simulink model "sim_real"  (R2016a)
settings: Solver=FixedStepAuto  StartTime=0.0  StopTime=25  RelTol=1e-3
InitFcn:
  | % Parametros
  | clear;
  | alpha1 = 0;
  | alpha2 = 120*pi/180;
  | alpha3 = 240*pi/180;
  | g = 9.8;
  | vs = 6e-10;
  | M = 1.83;
  | l1 = 0.09;
  | l2 = 0.09;
  | l3 = 0.09;
  | r1 = 0.072;
  | r2 = 0.072;
  | r3 = 0.072;
  | kt = 0.0059;
  | kem = 0.0059;
  | N = 19;
  | L = 0.00011;
  | R = 1.71;
  | Jm1 = 3.88e-7;
  | Jm2 = 3.88e-7;
  | Jm3 = 3.88e-7;
  | J1 = 8.1e-4;
  | J2 = 8.1e-4;
  | J3 = 8.1e-4;
  | J = 2.125;
  | eta = 0.83;
  | freq = 1000; % varia entre 2.5kHz e 5Mhz
  | mic = 0.46;
  | mis = 0.46;
  | sigma0 = 100;
  | sigma1 = 0.1;
  | sigma2 = 0.1;
  | 
  | mi = 0.25;
  | b = .1;
  | 
  | % Controlador
  | Kpx = 10;
  | Kix = 25;
  | Kpy = 10;
  | Kiy = 25;
  | Kvphi = 3;
  | Kpphi = 2.25;
  | 
  | kctr = kt*5.4*eta*N/(R*r1)
undefined symbols (not defined in the file or in its folder): magnitude
settings Model: MinMaxOverflowLogging=MinMaxAndOverflow  Creator=Pichau  LastModifiedBy=Pichau
settings DataIOCC: LimitDataPoints=on  MaxDataPoints=100000000  SaveFormat=Array  SignalLoggingSaveFormat=ModelDataLogs
settings OptimizationCC: OptimizeBlockIOStorage=off  BufferReuse=off  GlobalBufferReuse=off  ExpressionFolding=off  LocalBlockOutputs=off  RollThreshold=4
settings DebuggingCC: SaveWithParameterizedLinksMsg=none  UnderspecifiedInitializationDetection=Classic  MergeDetectMultiDrivingBlocksExec=none  SignalResolutionControl=TryResolveAllWithWarning  MultiTaskDSMMsg=warning  MultiTaskCondExecSysMsg=none
settings HardwareCC: ProdBitPerPointer=32  ProdLargestAtomicFloat=None  ProdIntDivRoundTo=Undefined  ProdEndianess=Unspecified  ProdWordSize=32  ProdHWDeviceType=32-bit Generic  TargetUnknown=on
settings ModelReferenceCC: PropagateSignalLabelsOutOfModel=off
settings GRTTargetCC: TargetFcnLib=ansi_tfl_tmw.mat  GeneratePreprocessorConditionals=Use local settings  CombineOutputUpdateFcns=off  GRTInterface=on
settings ConfigComp: CovModelRefEnable=Off

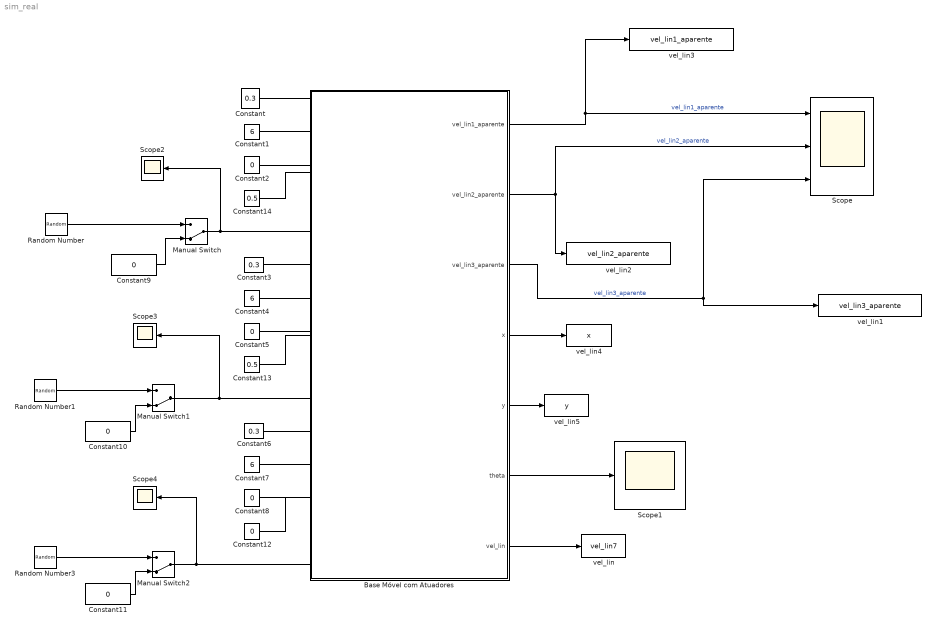
== system sim_real ==
  Base Móvel com Atuadores : Subsystem
  Constant : Constant  Value=0.3
  Constant1 : Constant  Value=6
  Constant{2,5,8..12} (7 alike) : Constant  Value=0
  Constant13 : Constant  Value=0.5
  Constant14 : Constant  Value=0.5
  Constant3 : Constant  Value=0.3
  Constant4 : Constant  Value=6
  Constant6 : Constant  Value=0.3
  Constant7 : Constant  Value=6
  Manual Switch : ManualSwitch  CurrentSetting=0
  Manual Switch1 : ManualSwitch  CurrentSetting=0
  Manual Switch2 : ManualSwitch  CurrentSetting=0
  Random Number : RandomNumber  Variance=0.003  Seed=123123  SampleTime=10
  Random Number1 : RandomNumber  Variance=0.003  Seed=2323  SampleTime=10
  Random Number3 : RandomNumber  Variance=0.003  Seed=55  SampleTime=10
  Scope : Scope  NumInputPorts=3
  Scope{1..4} (4 alike) : Scope
  vel_lin : ToWorkspace  VariableName=vel_lin7  SampleTime=0.01
  vel_lin1 : ToWorkspace  VariableName=vel_lin3_aparente  SampleTime=-1
  vel_lin2 : ToWorkspace  VariableName=vel_lin2_aparente  SampleTime=-1
  vel_lin3 : ToWorkspace  VariableName=vel_lin1_aparente  SampleTime=-1
  vel_lin4 : ToWorkspace  VariableName=x  SampleTime=-1
  vel_lin5 : ToWorkspace  VariableName=y  SampleTime=-1
  wires:
  Constant/1 -> ?
  Constant1/1 -> ?
  Constant2/1 -> ?
  Constant14/1 -> ?
  Constant9/1 -> Manual Switch/2
  Constant3/1 -> ?
  Constant4/1 -> ?
  Constant5/1 -> ?
  Constant13/1 -> ?
  Constant6/1 -> ?
  Constant7/1 -> ?
  Constant8/1 -> ?
  Constant12/1 -> ?
  Base Móvel com Atuadores/7(vel_lin) -> vel_lin/1
  Base Móvel com Atuadores/1(vel_lin1_aparente) -> vel_lin3/1, Scope/1  "vel_lin1_aparente"
  Base Móvel com Atuadores/2(vel_lin2_aparente) -> vel_lin2/1, Scope/2  "vel_lin2_aparente"
  Base Móvel com Atuadores/3(vel_lin3_aparente) -> vel_lin1/1, Scope/3  "vel_lin3_aparente"
  Base Móvel com Atuadores/6(theta) -> Scope1/1
  Base Móvel com Atuadores/5(y) -> vel_lin5/1
  Base Móvel com Atuadores/4(x) -> vel_lin4/1
  Random Number/1 -> Manual Switch/1
  Random Number1/1 -> Manual Switch1/1
  Manual Switch/1 -> Scope2/1
  Constant10/1 -> Manual Switch1/2
  Manual Switch1/1 -> Scope3/1
  Random Number3/1 -> Manual Switch2/1
  Constant11/1 -> Manual Switch2/2
  Manual Switch2/1 -> Scope4/1

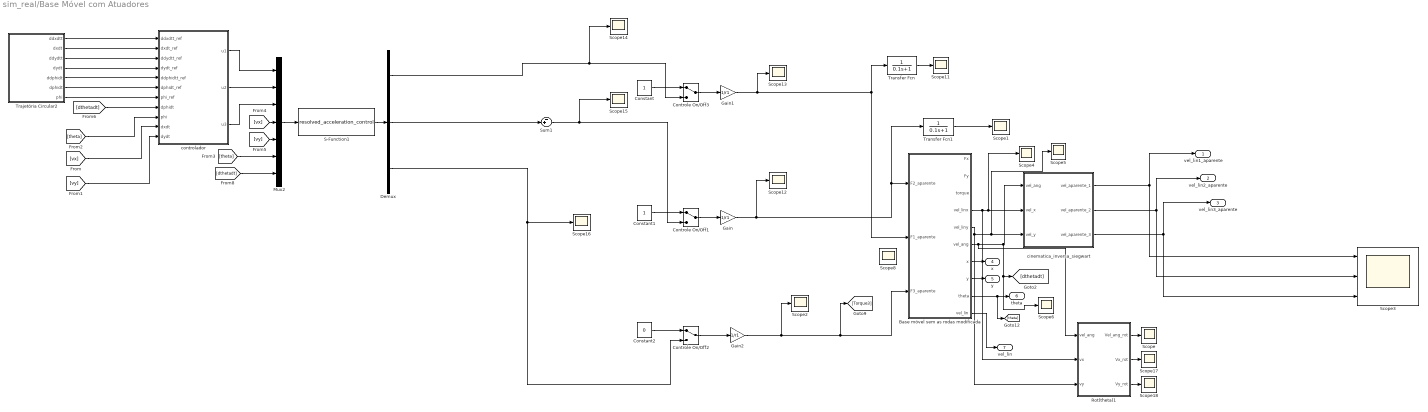
== system sim_real/Base Móvel com Atuadores ==
  Base móvel sem as rodas modificada : Subsystem
  Constant : Constant
  Constant1 : Constant
  Constant2 : Constant  Value=0
  Controle On/Off1 : ManualSwitch
  Controle On/Off2 : ManualSwitch
  Controle On/Off3 : ManualSwitch
  Demux : Demux  Outputs=3
  Gain : Gain  Gain=1/r1
  Gain1 : Gain  Gain=1/r1
  Gain2 : Gain  Gain=1/r1
  Mux2 : Mux  Inputs=7
  Rot(theta)1 : Subsystem
  S-Function1 : S-Function  FunctionName=resolved_acceleration_control  Parameters=r,L,m,J,Jw  SFunctionDeploymentMode=off  EnableBusSupport=off  mask{r=0.072, L=0.09, m=1.83, J=2.125, Jw=8.1e-4}
  Scope{,1..2,4..6,8,11..18} (15 alike) : Scope
  Scope3 : Scope  NumInputPorts=3
  Sum1 : Sum  Inputs=-+|
  Trajetória Circular2 : Subsystem
  Transfer Fcn : TransferFcn  Denominator=[0.1 1]
  Transfer Fcn1 : TransferFcn  Denominator=[0.1 1]
  cinematica_inversa_siegwart : Subsystem
  controlador : Subsystem
  vel_lin1_aparente : Outport
  vel_lin2_aparente : Outport  Port=2
  vel_lin3_aparente : Outport  Port=3
  x : Outport  Port=4
  y : Outport  Port=5
  theta : Outport  Port=6
  vel_lin : Outport  Port=7
  wires:
  cinematica_inversa_siegwart/1(vel_aparente_1) -> vel_lin1_aparente/1, Scope3/1
  Base móvel sem as rodas modificada/4(vel_linx) -> Rot(theta)1/2(vx), Scope4/1, cinematica_inversa_siegwart/2(vel_x)
  Controle On/Off3/1 -> Gain1/1
  cinematica_inversa_siegwart/2(vel_aparente_2) -> vel_lin2_aparente/1, Scope3/2
  cinematica_inversa_siegwart/3(vel_aparente_3) -> vel_lin3_aparente/1, Scope3/3
  Base móvel sem as rodas modificada/7(x) -> x/1
  Base móvel sem as rodas modificada/8(y) -> y/1
  Base móvel sem as rodas modificada/10(vel_lin) -> vel_lin/1
  Base móvel sem as rodas modificada/6(vel_ang) -> Rot(theta)1/1(vel_ang), cinematica_inversa_siegwart/1(vel_ang), [dthetadt], Scope6/1
  Transfer Fcn/1 -> Scope11/1
  Controle On/Off2/1 -> Gain2/1
  Transfer Fcn1/1 -> Scope1/1
  Constant/1 -> Controle On/Off3/1
  Constant1/1 -> Controle On/Off1/1
  Trajetória Circular2/2(dxdt) -> controlador/2(dxdt_ref)
  Trajetória Circular2/6(dphidt) -> controlador/6(dphidt_ref)
  Trajetória Circular2/1(ddxdtt) -> controlador/1(ddxdtt_ref)
  Trajetória Circular2/4(dydt) -> controlador/4(dydt_ref)
  Trajetória Circular2/3(ddydtt) -> controlador/3(ddydtt_ref)
  Trajetória Circular2/7(phi) -> controlador/7(phi_ref)
  Trajetória Circular2/5(ddphidt) -> controlador/5(ddphidtt_ref)
  controlador/1(u1) -> Mux2/1
  controlador/2(u2) -> Mux2/2
  controlador/3(u3) -> Mux2/3
  [vx] -> controlador/10(dxdt)
  [vy] -> controlador/11(dydt)
  [theta] -> controlador/9(phi)
  Mux2/1 -> S-Function1/1
  [theta] -> Mux2/6
  [vx] -> Mux2/4
  [vy] -> Mux2/5
  [dthetadt] -> controlador/8(dphidt)
  [dthetadt] -> Mux2/7
  S-Function1/1 -> Demux/1
  Demux/1 -> Scope14/1, Controle On/Off3/2
  Demux/3 -> Scope16/1, Controle On/Off2/2
  Demux/2 -> Sum1/2
  Controle On/Off1/1 -> Gain/1
  Sum1/1 -> Scope15/1, Controle On/Off1/2
  Base móvel sem as rodas modificada/9(theta) -> [theta], theta/1
  Gain/1 -> Scope12/1, Transfer Fcn1/1, Base móvel sem as rodas modificada/1(F2_aparente)
  Gain1/1 -> Scope13/1, Transfer Fcn/1, Base móvel sem as rodas modificada/2(F1_aparente)
  Gain2/1 -> Scope2/1, Base móvel sem as rodas modificada/3(F3_aparente), [Torque3]
  Rot(theta)1/2(Vx_rot) -> Scope17/1
  Rot(theta)1/3(Vy_rot) -> Scope18/1
  Rot(theta)1/1(Vel_ang_rot) -> Scope/1
  Constant2/1 -> Controle On/Off2/1
  Base móvel sem as rodas modificada/5(vel_liny) -> Rot(theta)1/3(vy), Scope5/1, cinematica_inversa_siegwart/3(vel_y)

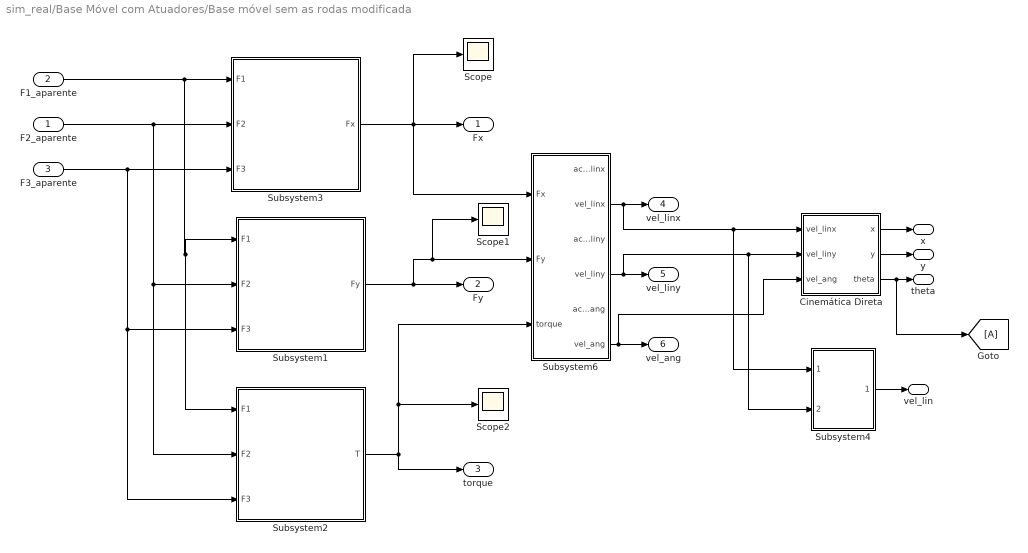
== system sim_real/Base Móvel com Atuadores/Base móvel sem as rodas modificada ==
  F2_aparente : Inport
  F1_aparente : Inport  Port=2
  F3_aparente : Inport  Port=3
  Cinemática Direta : Subsystem
  Scope : Scope
  Scope1 : Scope
  Scope2 : Scope
  Subsystem1 : Subsystem
  Subsystem2 : Subsystem
  Subsystem3 : Subsystem
  Subsystem4 : Subsystem
  Subsystem6 : Subsystem
  Fx : Outport
  Fy : Outport  Port=2
  torque : Outport  Port=3
  vel_linx : Outport  Port=4
  vel_liny : Outport  Port=5
  vel_ang : Outport  Port=6
  x : Outport  Port=7
  y : Outport  Port=8
  theta : Outport  Port=9
  vel_lin : Outport  Port=10
  wires:
  Subsystem3/1(Fx) -> Scope/1, Subsystem6/1(Fx), Fx/1
  Subsystem1/1(Fy) -> Scope1/1, Subsystem6/2(Fy), Fy/1
  F1_aparente/1 -> Subsystem2/1(F1), Subsystem1/1(F1), Subsystem3/1(F1)
  Subsystem6/2(vel_linx) -> vel_linx/1, Cinemática Direta/1(vel_linx), Subsystem4/1(vel_linx)
  Subsystem6/4(vel_liny) -> vel_liny/1, Cinemática Direta/2(vel_liny), Subsystem4/2(vel_liny)
  Subsystem6/6(vel_ang) -> vel_ang/1, Cinemática Direta/3(vel_ang)
  Subsystem2/1(T) -> torque/1, Subsystem6/3(torque), Scope2/1
  Cinemática Direta/1(x) -> x/1
  Cinemática Direta/2(y) -> y/1
  Cinemática Direta/3(theta) -> [A], theta/1
  Subsystem4/1(vel_lin) -> vel_lin/1
  F2_aparente/1 -> Subsystem2/2(F2), Subsystem1/2(F2), Subsystem3/2(F2)
  F3_aparente/1 -> Subsystem2/3(F3), Subsystem1/3(F3), Subsystem3/3(F3)

== system sim_real/Base Móvel com Atuadores/Rot(theta)1 ==
  vel_ang : Inport
  vx : Inport  Port=2
  vy : Inport  Port=3
  Integrator : Integrator
  Subsystem3 : Subsystem
  Subsystem4 : Subsystem
  Vel_ang_rot : Outport
  Vx_rot : Outport  Port=2
  Vy_rot : Outport  Port=3
  wires:
  Integrator/1 -> Subsystem3/1(theta), Subsystem4/1(theta)
  vel_ang/1 -> Integrator/1, Vel_ang_rot/1
  vy/1 -> Subsystem3/3(vy), Subsystem4/3(vy)
  vx/1 -> Subsystem3/2(vx), Subsystem4/2(vx)
  Subsystem4/1(vy_rot) -> Vy_rot/1
  Subsystem3/1(vx_rot) -> Vx_rot/1

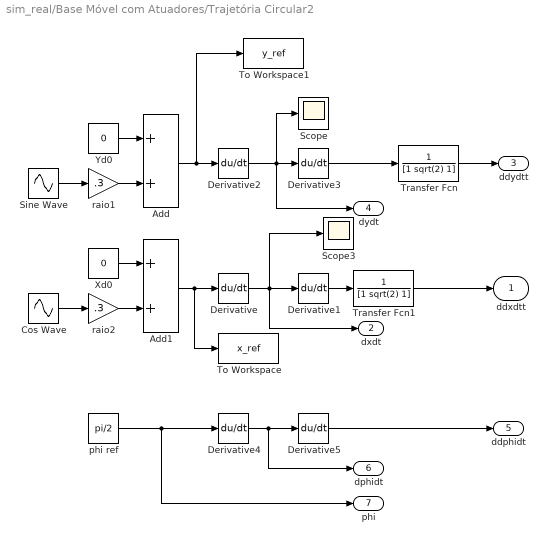
== system sim_real/Base Móvel com Atuadores/Trajetória Circular2 ==
  Add : Sum
  Add1 : Sum
  Cos Wave : Sin  Frequency=0.3  Phase=pi/2  SampleTime=0
  Derivative{,1..5} (6 alike) : Derivative
  Scope : Scope
  Scope3 : Scope
  Sine Wave : Sin  Frequency=0.3  SampleTime=0
  To Workspace : ToWorkspace  VariableName=x_ref  SaveFormat=Timeseries  SampleTime=-1
  To Workspace1 : ToWorkspace  VariableName=y_ref  SaveFormat=Timeseries  SampleTime=-1
  Transfer Fcn : TransferFcn  Denominator=[1 sqrt(2) 1]
  Transfer Fcn1 : TransferFcn  Denominator=[1 sqrt(2) 1]
  Xd0 : Constant  Value=0
  Yd0 : Constant  Value=0
  phi ref : Constant  Value=pi/2
  raio1 : Gain  Gain=.3
  raio2 : Gain  Gain=.3
  ddxdtt : Outport
  dxdt : Outport  Port=2
  ddydtt : Outport  Port=3
  dydt : Outport  Port=4
  ddphidt : Outport  Port=5
  dphidt : Outport  Port=6
  phi : Outport  Port=7
  wires:
  Transfer Fcn1/1 -> ddxdtt/1
  Transfer Fcn/1 -> ddydtt/1
  phi ref/1 -> Derivative4/1, phi/1
  Derivative5/1 -> ddphidt/1
  Derivative4/1 -> Derivative5/1, dphidt/1
  Derivative1/1 -> Transfer Fcn1/1
  Derivative3/1 -> Transfer Fcn/1
  Derivative2/1 -> Derivative3/1, Scope/1, dydt/1
  Derivative/1 -> Scope3/1, Derivative1/1, dxdt/1
  Sine Wave/1 -> raio1/1
  raio1/1 -> Add/2
  Add/1 -> To Workspace1/1, Derivative2/1
  Add1/1 -> To Workspace/1, Derivative/1
  raio2/1 -> Add1/2
  Cos Wave/1 -> raio2/1
  Xd0/1 -> Add1/1
  Yd0/1 -> Add/1

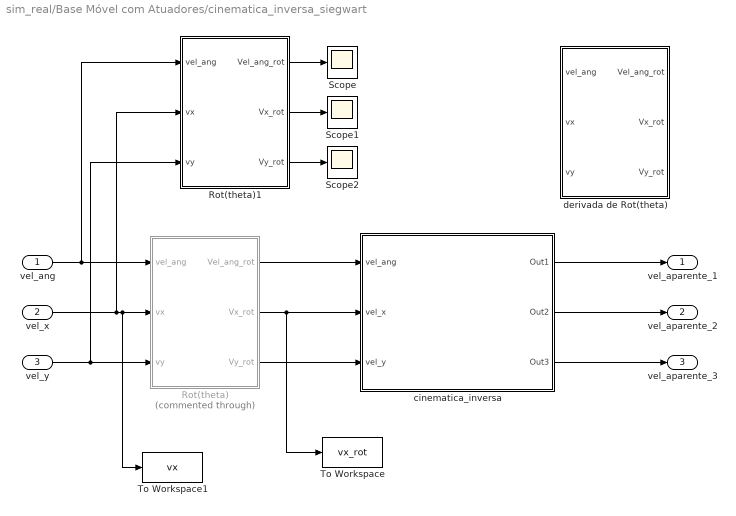
== system sim_real/Base Móvel com Atuadores/cinematica_inversa_siegwart ==
  vel_ang : Inport
  vel_x : Inport  Port=2
  vel_y : Inport  Port=3
  Rot(theta) : Subsystem  Commented=through
  Rot(theta)1 : Subsystem
  Scope : Scope
  Scope1 : Scope
  Scope2 : Scope
  To Workspace : ToWorkspace  VariableName=vx_rot  SampleTime=-1
      settings: Save2DSignal=2-D array (concatenate along first dimension)
  To Workspace1 : ToWorkspace  VariableName=vx  SampleTime=-1
      settings: Save2DSignal=2-D array (concatenate along first dimension)
  cinematica_inversa : Subsystem
  derivada de Rot(theta) : Subsystem
  vel_aparente_1 : Outport
  vel_aparente_2 : Outport  Port=2
  vel_aparente_3 : Outport  Port=3
  wires:
  vel_x/1 -> Rot(theta)1/2(vx), To Workspace1/1, Rot(theta)/2(vx)
  vel_y/1 -> Rot(theta)1/3(vy), Rot(theta)/3(vy)
  Rot(theta)/2(Vx_rot) -> To Workspace/1, cinematica_inversa/2(vel_x)
  Rot(theta)/3(Vy_rot) -> cinematica_inversa/3(vel_y)
  Rot(theta)/1(Vel_ang_rot) -> cinematica_inversa/1(vel_ang)
  cinematica_inversa/1(Out1) -> vel_aparente_1/1
  cinematica_inversa/2(Out2) -> vel_aparente_2/1
  cinematica_inversa/3(Out3) -> vel_aparente_3/1
  vel_ang/1 -> Rot(theta)1/1(vel_ang), Rot(theta)/1(vel_ang)
  Rot(theta)1/1(Vel_ang_rot) -> Scope/1
  Rot(theta)1/2(Vx_rot) -> Scope1/1
  Rot(theta)1/3(Vy_rot) -> Scope2/1

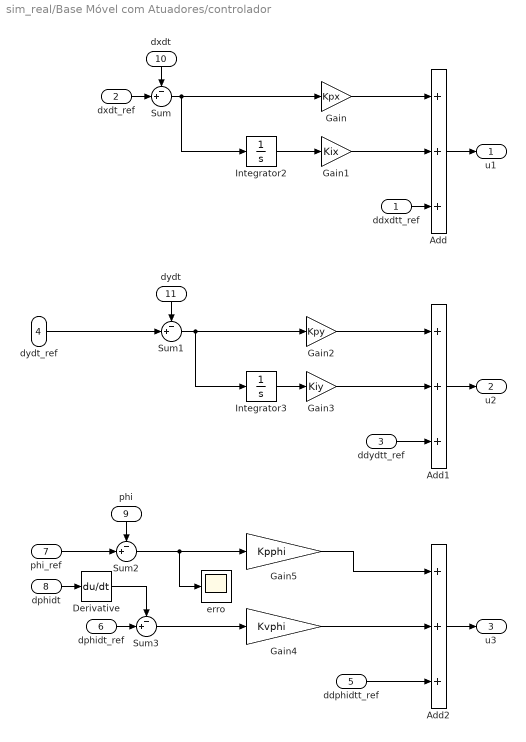
== system sim_real/Base Móvel com Atuadores/controlador ==
  ddxdtt_ref : Inport
  dxdt_ref : Inport  Port=2
  ddydtt_ref : Inport  Port=3
  dydt_ref : Inport  Port=4
  ddphidtt_ref : Inport  Port=5
  dphidt_ref : Inport  Port=6
  phi_ref : Inport  Port=7
  dphidt : Inport  Port=8
  phi : Inport  Port=9
  dxdt : Inport  Port=10
  dydt : Inport  Port=11
  Add : Sum  Inputs=+++
  Add1 : Sum  Inputs=+++
  Add2 : Sum  Inputs=+++
  Derivative : Derivative
  Gain : Gain  Gain=Kpx
  Gain1 : Gain  Gain=Kix
  Gain2 : Gain  Gain=Kpy
  Gain3 : Gain  Gain=Kiy
  Gain4 : Gain  Gain=Kvphi
  Gain5 : Gain  Gain=Kpphi
  Integrator2 : Integrator
  Integrator3 : Integrator
  Sum{,1..3} (4 alike) : Sum  Inputs=-+|
  erro : Scope
  u1 : Outport
  u2 : Outport  Port=2
  u3 : Outport  Port=3
  wires:
  Sum2/1 -> Gain5/1, erro/1
  Sum1/1 -> Gain2/1, Integrator3/1
  Gain1/1 -> Add/2
  Integrator2/1 -> Gain1/1
  dydt_ref/1 -> Sum1/2
  Add/1 -> u1/1
  Gain2/1 -> Add1/1
  Integrator3/1 -> Gain3/1
  Derivative/1 -> Sum3/1
  Gain4/1 -> Add2/2
  Sum/1 -> Gain/1, Integrator2/1
  Gain3/1 -> Add1/2
  Gain5/1 -> Add2/1
  Sum3/1 -> Gain4/1
  ddphidtt_ref/1 -> Add2/3
  ddydtt_ref/1 -> Add1/3
  Add1/1 -> u2/1
  ddxdtt_ref/1 -> Add/3
  phi/1 -> Sum2/1
  Add2/1 -> u3/1
  dxdt_ref/1 -> Sum/2
  dxdt/1 -> Sum/1
  phi_ref/1 -> Sum2/2
  Gain/1 -> Add/1
  dydt/1 -> Sum1/1
  dphidt/1 -> Derivative/1
  dphidt_ref/1 -> Sum3/2

== system sim_real/Base Móvel com Atuadores/Base móvel sem as rodas modificada/Cinemática Direta ==
  vel_linx : Inport
  vel_liny : Inport  Port=2
  vel_ang : Inport  Port=3
  Integrator1 : Integrator  UpperSaturationLimit=1e-6  LowerSaturationLimit=-1e-6
  Integrator3 : Integrator  UpperSaturationLimit=1e-6  LowerSaturationLimit=-1e-6
  Integrator4 : Integrator  UpperSaturationLimit=1e-6  LowerSaturationLimit=-1e-6
  x : Outport
  y : Outport  Port=2
  theta : Outport  Port=3
  wires:
  Integrator4/1 -> y/1
  Integrator3/1 -> x/1
  vel_linx/1 -> Integrator3/1
  vel_liny/1 -> Integrator4/1
  vel_ang/1 -> Integrator1/1
  Integrator1/1 -> theta/1

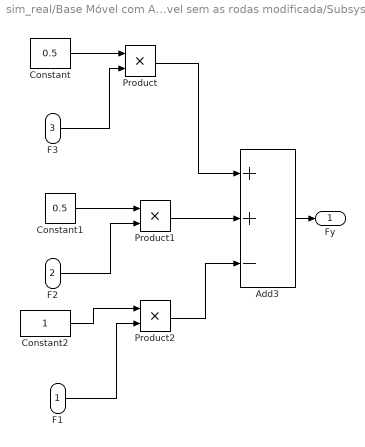
== system sim_real/Base Móvel com Atuadores/Base móvel sem as rodas modificada/Subsystem1 ==
  F1 : Inport
  F2 : Inport  Port=2
  F3 : Inport  Port=3
  Add3 : Sum  Inputs=++-
  Constant : Constant  Value=0.5
  Constant1 : Constant  Value=0.5
  Constant2 : Constant
  Product : Product
  Product1 : Product
  Product2 : Product
  Fy : Outport
  wires:
  Product2/1 -> Add3/3
  Product/1 -> Add3/1
  Constant2/1 -> Product2/1
  Constant1/1 -> Product1/1
  Product1/1 -> Add3/2
  Constant/1 -> Product/1
  F2/1 -> Product1/2
  F1/1 -> Product2/2
  F3/1 -> Product/2
  Add3/1 -> Fy/1

== system sim_real/Base Móvel com Atuadores/Base móvel sem as rodas modificada/Subsystem2 ==
  F1 : Inport
  F2 : Inport  Port=2
  F3 : Inport  Port=3
  Add3 : Sum  Inputs=---
  Constant : Constant  Value=0.09
  Constant1 : Constant  Value=0.09
  Constant2 : Constant  Value=0.09
  Product : Product
  Product1 : Product
  Product2 : Product
  T : Outport
  wires:
  Add3/1 -> T/1
  F3/1 -> Product/2
  F1/1 -> Product2/2
  F2/1 -> Product1/2
  Constant/1 -> Product/1
  Product1/1 -> Add3/2
  Constant1/1 -> Product1/1
  Constant2/1 -> Product2/1
  Product/1 -> Add3/1
  Product2/1 -> Add3/3

== system sim_real/Base Móvel com Atuadores/Base móvel sem as rodas modificada/Subsystem3 ==
  F1 : Inport
  F2 : Inport  Port=2
  F3 : Inport  Port=3
  Add3 : Sum  Inputs=-++
  Constant : Constant  Value=0.8660
  Constant1 : Constant  Value=0.8660
  Constant2 : Constant  Value=0
  Product : Product
  Product1 : Product
  Product2 : Product
  Fx : Outport
  wires:
  Add3/1 -> Fx/1
  F3/1 -> Product/2
  F1/1 -> Product2/2
  F2/1 -> Product1/2
  Constant/1 -> Product/1
  Product1/1 -> Add3/2
  Constant1/1 -> Product1/1
  Constant2/1 -> Product2/1
  Product/1 -> Add3/1
  Product2/1 -> Add3/3

== system sim_real/Base Móvel com Atuadores/Base móvel sem as rodas modificada/Subsystem4 ==
  vel_linx : Inport
  vel_liny : Inport  Port=2
  Math Function : Math  Operator=magnitude^2  SaturateOnIntegerOverflow=on
  Math Function1 : Math  Operator=magnitude^2  SaturateOnIntegerOverflow=on
  Math Function2 : Math  Operator=sqrt  SaturateOnIntegerOverflow=on
  Sum15 : Sum  Inputs=|++
  vel_lin : Outport
  wires:
  Math Function/1 -> Sum15/1
  Math Function1/1 -> Sum15/2
  Sum15/1 -> Math Function2/1
  vel_linx/1 -> Math Function/1
  vel_liny/1 -> Math Function1/1
  Math Function2/1 -> vel_lin/1

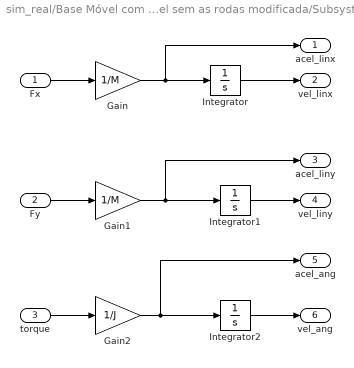
== system sim_real/Base Móvel com Atuadores/Base móvel sem as rodas modificada/Subsystem6 ==
  Fx : Inport
  Fy : Inport  Port=2
  torque : Inport  Port=3
  Gain : Gain  Gain=1/M
  Gain1 : Gain  Gain=1/M
  Gain2 : Gain  Gain=1/J
  Integrator : Integrator  UpperSaturationLimit=1e-6  LowerSaturationLimit=-1e-6
  Integrator1 : Integrator  UpperSaturationLimit=1e-6  LowerSaturationLimit=-1e-6
  Integrator2 : Integrator  UpperSaturationLimit=1e-6  LowerSaturationLimit=-1e-6
  acel_linx : Outport
  vel_linx : Outport  Port=2
  acel_liny : Outport  Port=3
  vel_liny : Outport  Port=4
  acel_ang : Outport  Port=5
  vel_ang : Outport  Port=6
  wires:
  Gain/1 -> acel_linx/1, Integrator/1
  Gain1/1 -> Integrator1/1, acel_liny/1
  Gain2/1 -> Integrator2/1, acel_ang/1
  Fx/1 -> Gain/1
  Integrator/1 -> vel_linx/1
  Integrator1/1 -> vel_liny/1
  torque/1 -> Gain2/1
  Integrator2/1 -> vel_ang/1
  Fy/1 -> Gain1/1

== system sim_real/Base Móvel com Atuadores/Rot(theta)1/Subsystem3 ==
  theta : Inport
  vx : Inport  Port=2
  vy : Inport  Port=3
  Add : Sum
  Divide : Product  Inputs=**
  Divide1 : Product  Inputs=**
  Trigonometric Function : Trigonometry
  Trigonometric Function1 : Trigonometry  Operator=cos
  vx_rot : Outport
  wires:
  vx/1 -> Divide/2
  vy/1 -> Divide1/2
  Trigonometric Function1/1 -> Divide/1
  Divide1/1 -> Add/2
  Add/1 -> vx_rot/1
  theta/1 -> Trigonometric Function/1, Trigonometric Function1/1
  Trigonometric Function/1 -> Divide1/1
  Divide/1 -> Add/1

== system sim_real/Base Móvel com Atuadores/Rot(theta)1/Subsystem4 ==
  theta : Inport
  vx : Inport  Port=2
  vy : Inport  Port=3
  Add : Sum  Inputs=-+
  Divide : Product  Inputs=**
  Divide1 : Product  Inputs=**
  Trigonometric Function : Trigonometry  Operator=cos
  Trigonometric Function1 : Trigonometry
  vy_rot : Outport
  wires:
  Divide/1 -> Add/1
  Trigonometric Function/1 -> Divide1/1
  theta/1 -> Trigonometric Function1/1, Trigonometric Function/1
  Add/1 -> vy_rot/1
  Divide1/1 -> Add/2
  Trigonometric Function1/1 -> Divide/1
  vy/1 -> Divide1/2
  vx/1 -> Divide/2

== system sim_real/Base Móvel com Atuadores/cinematica_inversa_siegwart/Rot(theta) ==
  vel_ang : Inport
  vx : Inport  Port=2
  vy : Inport  Port=3
  Integrator : Integrator
  Subsystem3 : Subsystem
  Subsystem4 : Subsystem
  Vel_ang_rot : Outport
  Vx_rot : Outport  Port=2
  Vy_rot : Outport  Port=3
  wires:
  Subsystem3/1(vx_rot) -> Vx_rot/1
  Subsystem4/1(vy_rot) -> Vy_rot/1
  vx/1 -> Subsystem4/2(vx), Subsystem3/2(vx)
  vy/1 -> Subsystem4/3(vy), Subsystem3/3(vy)
  vel_ang/1 -> Vel_ang_rot/1, Integrator/1
  Integrator/1 -> Subsystem4/1(theta), Subsystem3/1(theta)

== system sim_real/Base Móvel com Atuadores/cinematica_inversa_siegwart/Rot(theta)1 ==
  vel_ang : Inport
  vx : Inport  Port=2
  vy : Inport  Port=3
  Integrator : Integrator
  Subsystem3 : Subsystem
  Subsystem4 : Subsystem
  Vel_ang_rot : Outport
  Vx_rot : Outport  Port=2
  Vy_rot : Outport  Port=3
  wires:
  Integrator/1 -> Subsystem3/1(theta), Subsystem4/1(theta)
  vel_ang/1 -> Integrator/1, Vel_ang_rot/1
  vy/1 -> Subsystem3/3(vy), Subsystem4/3(vy)
  vx/1 -> Subsystem3/2(vx), Subsystem4/2(vx)
  Subsystem4/1(vy_rot) -> Vy_rot/1
  Subsystem3/1(vx_rot) -> Vx_rot/1

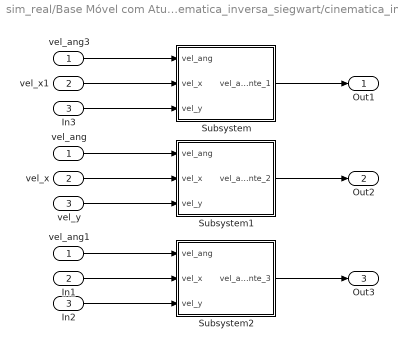
== system sim_real/Base Móvel com Atuadores/cinematica_inversa_siegwart/cinematica_inversa ==
  vel_ang : Inport
  vel_x : Inport  Port=2
  vel_y : Inport  Port=3
  In1 : InportShadow  Port=2
  In2 : InportShadow  Port=3
  In3 : InportShadow  Port=3
  Subsystem : Subsystem
  Subsystem1 : Subsystem
  Subsystem2 : Subsystem
  vel_ang1 : InportShadow
  vel_ang3 : InportShadow
  vel_x1 : InportShadow  Port=2
  Out1 : Outport
  Out2 : Outport  Port=2
  Out3 : Outport  Port=3
  wires:
  Subsystem/1(vel_aparente_1) -> Out1/1
  vel_x/1 -> Subsystem1/2(vel_x)
  vel_ang/1 -> Subsystem1/1(vel_ang)
  vel_y/1 -> Subsystem1/3(vel_y)
  Subsystem1/1(vel_aparente_2) -> Out2/1
  Subsystem2/1(vel_aparente_3) -> Out3/1
  vel_ang3/1 -> Subsystem/1(vel_ang)
  vel_x1/1 -> Subsystem/2(vel_x)
  vel_ang1/1 -> Subsystem2/1(vel_ang)
  In1/1 -> Subsystem2/2(vel_x)
  In2/1 -> Subsystem2/3(vel_y)
  In3/1 -> Subsystem/3(vel_y)

== system sim_real/Base Móvel com Atuadores/cinematica_inversa_siegwart/derivada de Rot(theta) ==
  vel_ang : Inport
  vx : Inport  Port=2
  vy : Inport  Port=3
  Integrator : Integrator
  Subsystem3 : Subsystem
  Subsystem4 : Subsystem
  Vel_ang_rot : Outport
  Vx_rot : Outport  Port=2
  Vy_rot : Outport  Port=3
  wires:
  Subsystem3/1(vx_rot) -> Vx_rot/1
  Subsystem4/1(vy_rot) -> Vy_rot/1
  vx/1 -> Subsystem4/2(vx), Subsystem3/2(vx)
  vy/1 -> Subsystem4/3(vy), Subsystem3/3(vy)
  vel_ang/1 -> Vel_ang_rot/1, Integrator/1
  Integrator/1 -> Subsystem4/1(theta), Subsystem3/1(theta)

== system sim_real/Base Móvel com Atuadores/cinematica_inversa_siegwart/Rot(theta)/Subsystem3 ==
  theta : Inport
  vx : Inport  Port=2
  vy : Inport  Port=3
  Add : Sum
  Divide : Product  Inputs=**
  Divide1 : Product  Inputs=**
  Trigonometric Function : Trigonometry
  Trigonometric Function1 : Trigonometry  Operator=cos
  vx_rot : Outport
  wires:
  Divide/1 -> Add/1
  Trigonometric Function/1 -> Divide1/1
  theta/1 -> Trigonometric Function1/1, Trigonometric Function/1
  Add/1 -> vx_rot/1
  Divide1/1 -> Add/2
  Trigonometric Function1/1 -> Divide/1
  vy/1 -> Divide1/2
  vx/1 -> Divide/2

== system sim_real/Base Móvel com Atuadores/cinematica_inversa_siegwart/Rot(theta)/Subsystem4 ==
  theta : Inport
  vx : Inport  Port=2
  vy : Inport  Port=3
  Add : Sum  Inputs=-+
  Divide : Product  Inputs=**
  Divide1 : Product  Inputs=**
  Trigonometric Function : Trigonometry  Operator=cos
  Trigonometric Function1 : Trigonometry
  vy_rot : Outport
  wires:
  vx/1 -> Divide/2
  vy/1 -> Divide1/2
  Trigonometric Function1/1 -> Divide/1
  Divide1/1 -> Add/2
  Add/1 -> vy_rot/1
  theta/1 -> Trigonometric Function/1, Trigonometric Function1/1
  Trigonometric Function/1 -> Divide1/1
  Divide/1 -> Add/1

== system sim_real/Base Móvel com Atuadores/cinematica_inversa_siegwart/Rot(theta)1/Subsystem3 ==
  theta : Inport
  vx : Inport  Port=2
  vy : Inport  Port=3
  Add : Sum
  Divide : Product  Inputs=**
  Divide1 : Product  Inputs=**
  Trigonometric Function : Trigonometry
  Trigonometric Function1 : Trigonometry  Operator=cos
  vx_rot : Outport
  wires:
  vx/1 -> Divide/2
  vy/1 -> Divide1/2
  Trigonometric Function1/1 -> Divide/1
  Divide1/1 -> Add/2
  Add/1 -> vx_rot/1
  theta/1 -> Trigonometric Function/1, Trigonometric Function1/1
  Trigonometric Function/1 -> Divide1/1
  Divide/1 -> Add/1

== system sim_real/Base Móvel com Atuadores/cinematica_inversa_siegwart/Rot(theta)1/Subsystem4 ==
  theta : Inport
  vx : Inport  Port=2
  vy : Inport  Port=3
  Add : Sum  Inputs=-+
  Divide : Product  Inputs=**
  Divide1 : Product  Inputs=**
  Trigonometric Function : Trigonometry  Operator=cos
  Trigonometric Function1 : Trigonometry
  vy_rot : Outport
  wires:
  Divide/1 -> Add/1
  Trigonometric Function/1 -> Divide1/1
  theta/1 -> Trigonometric Function1/1, Trigonometric Function/1
  Add/1 -> vy_rot/1
  Divide1/1 -> Add/2
  Trigonometric Function1/1 -> Divide/1
  vy/1 -> Divide1/2
  vx/1 -> Divide/2

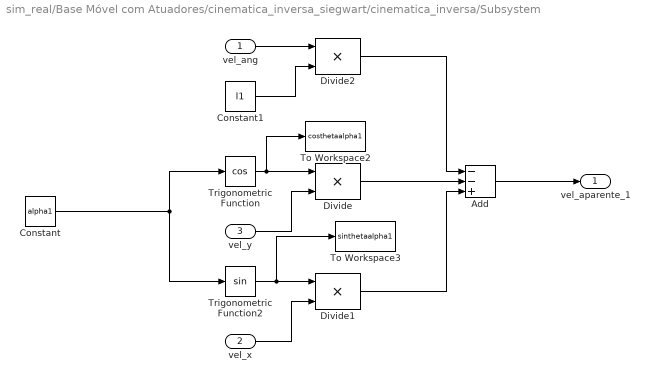
== system sim_real/Base Móvel com Atuadores/cinematica_inversa_siegwart/cinematica_inversa/Subsystem ==
  vel_ang : Inport
  vel_x : Inport  Port=2
  vel_y : Inport  Port=3
  Add : Sum  Inputs=--+
  Constant : Constant  Value=alpha1
  Constant1 : Constant  Value=l1
  Divide : Product  Inputs=**
  Divide1 : Product  Inputs=**
  Divide2 : Product  Inputs=**
  To Workspace2 : ToWorkspace  VariableName=costhetaalpha1  SampleTime=-1
      settings: Save2DSignal=2-D array (concatenate along first dimension)
  To Workspace3 : ToWorkspace  VariableName=sinthetaalpha1  SampleTime=-1
      settings: Save2DSignal=2-D array (concatenate along first dimension)
  Trigonometric Function : Trigonometry  Operator=cos
  Trigonometric Function2 : Trigonometry
  vel_aparente_1 : Outport
  wires:
  vel_y/1 -> Divide/2
  vel_ang/1 -> Divide2/1
  Trigonometric Function/1 -> To Workspace2/1, Divide/1
  Constant/1 -> Trigonometric Function/1, Trigonometric Function2/1
  Trigonometric Function2/1 -> To Workspace3/1, Divide1/1
  vel_x/1 -> Divide1/2
  Divide/1 -> Add/2
  Divide1/1 -> Add/3
  Constant1/1 -> Divide2/2
  Divide2/1 -> Add/1
  Add/1 -> vel_aparente_1/1

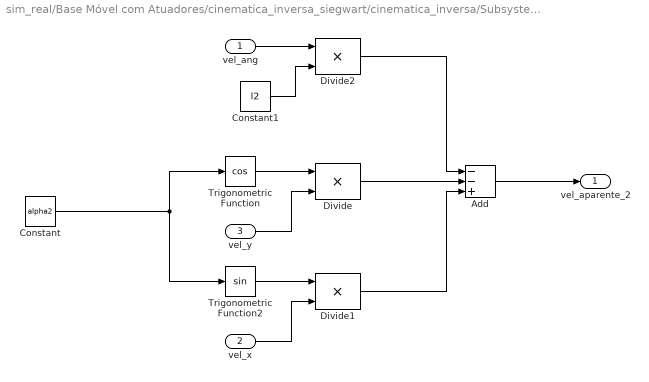
== system sim_real/Base Móvel com Atuadores/cinematica_inversa_siegwart/cinematica_inversa/Subsystem1 ==
  vel_ang : Inport
  vel_x : Inport  Port=2
  vel_y : Inport  Port=3
  Add : Sum  Inputs=--+
  Constant : Constant  Value=alpha2
  Constant1 : Constant  Value=l2
  Divide : Product  Inputs=**
  Divide1 : Product  Inputs=**
  Divide2 : Product  Inputs=**
  Trigonometric Function : Trigonometry  Operator=cos
  Trigonometric Function2 : Trigonometry
  vel_aparente_2 : Outport
  wires:
  Add/1 -> vel_aparente_2/1
  Divide2/1 -> Add/1
  Constant1/1 -> Divide2/2
  Divide1/1 -> Add/3
  Divide/1 -> Add/2
  vel_x/1 -> Divide1/2
  Trigonometric Function2/1 -> Divide1/1
  Constant/1 -> Trigonometric Function2/1, Trigonometric Function/1
  Trigonometric Function/1 -> Divide/1
  vel_ang/1 -> Divide2/1
  vel_y/1 -> Divide/2

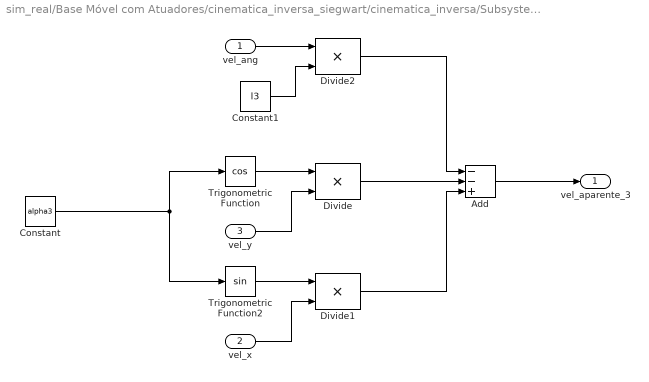
== system sim_real/Base Móvel com Atuadores/cinematica_inversa_siegwart/cinematica_inversa/Subsystem2 ==
  vel_ang : Inport
  vel_x : Inport  Port=2
  vel_y : Inport  Port=3
  Add : Sum  Inputs=--+
  Constant : Constant  Value=alpha3
  Constant1 : Constant  Value=l3
  Divide : Product  Inputs=**
  Divide1 : Product  Inputs=**
  Divide2 : Product  Inputs=**
  Trigonometric Function : Trigonometry  Operator=cos
  Trigonometric Function2 : Trigonometry
  vel_aparente_3 : Outport
  wires:
  vel_y/1 -> Divide/2
  vel_ang/1 -> Divide2/1
  Trigonometric Function/1 -> Divide/1
  Constant/1 -> Trigonometric Function/1, Trigonometric Function2/1
  Trigonometric Function2/1 -> Divide1/1
  vel_x/1 -> Divide1/2
  Divide/1 -> Add/2
  Divide1/1 -> Add/3
  Constant1/1 -> Divide2/2
  Divide2/1 -> Add/1
  Add/1 -> vel_aparente_3/1

== system sim_real/Base Móvel com Atuadores/cinematica_inversa_siegwart/derivada de Rot(theta)/Subsystem3 ==
  theta : Inport
  vx : Inport  Port=2
  vy : Inport  Port=3
  Add : Sum
  Divide : Product  Inputs=**
  Divide1 : Product  Inputs=**
  Trigonometric Function : Trigonometry
  Trigonometric Function1 : Trigonometry  Operator=cos
  vx_rot : Outport
  wires:
  Divide/1 -> Add/1
  Trigonometric Function/1 -> Divide1/1
  theta/1 -> Trigonometric Function1/1, Trigonometric Function/1
  Add/1 -> vx_rot/1
  Divide1/1 -> Add/2
  Trigonometric Function1/1 -> Divide/1
  vy/1 -> Divide1/2
  vx/1 -> Divide/2

== system sim_real/Base Móvel com Atuadores/cinematica_inversa_siegwart/derivada de Rot(theta)/Subsystem4 ==
  theta : Inport
  vx : Inport  Port=2
  vy : Inport  Port=3
  Add : Sum  Inputs=-+
  Divide : Product  Inputs=**
  Divide1 : Product  Inputs=**
  Trigonometric Function : Trigonometry  Operator=cos
  Trigonometric Function1 : Trigonometry
  vy_rot : Outport
  wires:
  vx/1 -> Divide/2
  vy/1 -> Divide1/2
  Trigonometric Function1/1 -> Divide/1
  Divide1/1 -> Add/2
  Add/1 -> vy_rot/1
  theta/1 -> Trigonometric Function/1, Trigonometric Function1/1
  Trigonometric Function/1 -> Divide1/1
  Divide/1 -> Add/1
